simulink model "MagLevLinearModel"  (R2015b)
settings: Solver=VariableStepAuto  StartTime=0.0  StopTime=10.0  RelTol=1e-3
values from neighbouring files (symbols this model uses):
  delta_V = V-v_o    [LinearModelVsNonLinearModel.m]
  i_o = 1.0005    [LinearModelVsNonLinearModel.m]
  Km = 6.5308*10^-5    (= 6.5308e-05)    [LinearModelVsNonLinearModel.m]
  L = 0.4125    [LinearModelVsNonLinearModel.m]
  Mb = 0.068    [LinearModelVsNonLinearModel.m]
  Rc = 10    [LinearModelVsNonLinearModel.m]
  Rs = 1    [LinearModelVsNonLinearModel.m]
  v_o = 11.0055    [LinearModelVsNonLinearModel.m]
  x_o = 0.007    [LinearModelVsNonLinearModel.m]
settings Model: Creator=Christopher  LastModifiedBy=Christopher
settings ConfigComp: CovModelRefEnable=Off

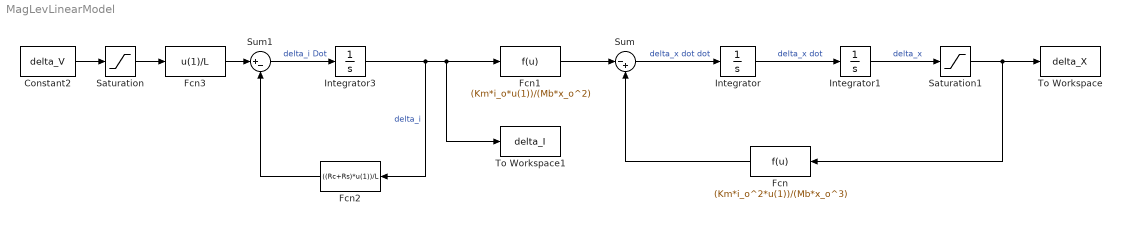
== system MagLevLinearModel ==
  Constant2 : Constant  Value=delta_V
  Fcn : Fcn  Expr=(Km*i_o^2*u(1))/(Mb*x_o^3)
  Fcn1 : Fcn  Expr=(Km*i_o*u(1))/(Mb*x_o^2)
  Fcn2 : Fcn  Expr=((Rc+Rs)*u(1))/L
  Fcn3 : Fcn  Expr=u(1)/L
  Integrator : Integrator  InitialCondition=0-x_o
  Integrator1 : Integrator  InitialCondition=0.014-x_o
  Integrator3 : Integrator  InitialCondition=0-i_o
  Saturation : Saturate  UpperLimit=24-v_o  LowerLimit=-24-v_o
  Saturation1 : Saturate  UpperLimit=0.014-x_o  LowerLimit=0.00001-x_o
  Sum : Sum  Inputs=|-+
  Sum1 : Sum  Inputs=|+-
  To Workspace : ToWorkspace  VariableName=delta_X  SaveFormat=Structure With Time  SampleTime=-1
  To Workspace1 : ToWorkspace  VariableName=delta_I  SaveFormat=Structure With Time  SampleTime=-1
  wires:
  Sum/1 -> Integrator/1  "delta_x dot dot"
  Integrator/1 -> Integrator1/1  "delta_x dot"
  Integrator1/1 -> Saturation1/1  "delta_x"
  Fcn/1 -> Sum/2
  Fcn1/1 -> Sum/1
  Fcn3/1 -> Sum1/1
  Sum1/1 -> Integrator3/1  "delta_i Dot"
  Integrator3/1 -> To Workspace1/1, Fcn1/1, Fcn2/1  "delta_i"
  Fcn2/1 -> Sum1/2
  Saturation1/1 -> To Workspace/1, Fcn/1
  Saturation/1 -> Fcn3/1
  Constant2/1 -> Saturation/1
